simulink model "SimuLanzador"  (R2020b)
settings: Solver=VariableStepAuto  StartTime=0.0  StopTime=300  RelTol=1e-3
model workspace (MAT data in the model file):
  Ang0 = [0; 0; 0]
  VelAng0 = [0; 0; 0]
  altura = 3.5
  delta = 0.05
  mu = 0.01
  r = 2.25
  radio = 2.25
libraries: simulink_extras x5, sharedutil x5, sharedtransform x3, aerolibutil x2, aerolibbdyn x2, vrlib x1, simulink x1
settings Model: Creator=Sergio  LastModifiedBy=Sergio
settings SolverCC: ZeroCrossAlgorithm=Adaptive  AlgebraicLoopSolver=LineSearch

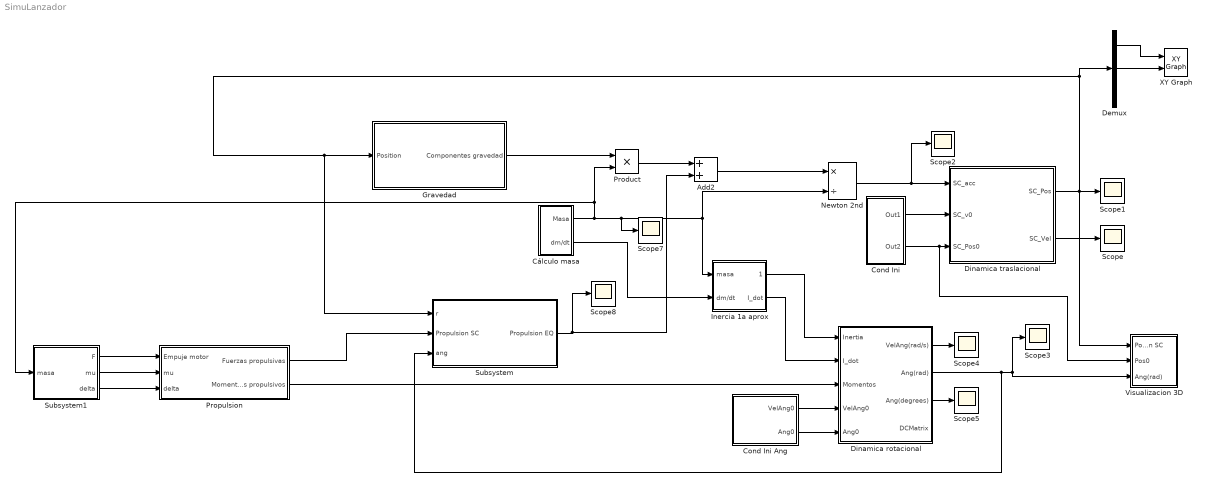
== system SimuLanzador ==
  Add2 : Sum
  Cond Ini : Subsystem  mask{v0=[0,0,0], Pos0=[1737100,0,0]}
  Cond Ini Ang : Subsystem  mask{VelAng0=[0,0,0], Ang0=[0,0,0]}
  Cálculo masa : Subsystem
  Demux : Demux  Outputs=3
  Dinamica rotacional : Subsystem
  Dinamica traslacional : Subsystem
  Gravedad : Subsystem
  Inercia 1a aprox : Subsystem
  Newton 2nd : Product  Inputs=*/
  Product : Product
  Propulsion : Subsystem
  Scope{,1..5,7..8} (8 alike) : Scope
  Subsystem : Subsystem
  Subsystem1 : Subsystem
  Visualizacion 3D : Subsystem
  XY Graph : simulink/Sinks/XY Graph  xmin=-2500000  xmax=2500000  ymin=-2500000  ymax=2500000  st=-1
  wires:
  Cond Ini/1(Out1) -> Dinamica traslacional/2(SC_v0)
  Cond Ini/2(Out2) -> Visualizacion 3D/2(Pos0), Dinamica traslacional/3(SC_Pos0)
  Newton 2nd/1 -> Scope2/1, Dinamica traslacional/1(SC_acc)
  Dinamica traslacional/2(SC_Vel) -> Scope/1
  Inercia 1a aprox/1(Inertia) -> Dinamica rotacional/1(Inertia)
  Dinamica rotacional/1(VelAng(rad/s)) -> Scope4/1
  Cond Ini Ang/1(VelAng0) -> Dinamica rotacional/4(VelAng0)
  Dinamica rotacional/3(Ang(degrees)) -> Scope5/1
  Product/1 -> Add2/1
  Gravedad/1(Componentes gravedad) -> Product/1
  Add2/1 -> Newton 2nd/1
  Subsystem/1(Propulsion EQ) -> Add2/2, Scope8/1
  Dinamica rotacional/2(Ang(rad)) -> Subsystem/3(ang), Scope3/1, Visualizacion 3D/3(Ang(rad))
  Inercia 1a aprox/2(I_dot) -> Dinamica rotacional/2(I_dot)
  Cálculo masa/2(dm/dt) -> Inercia 1a aprox/2(dm/dt)
  Cálculo masa/1(Masa) -> Scope7/1, Inercia 1a aprox/1(masa), Newton 2nd/2, Subsystem1/1(masa), Product/2
  Subsystem1/1(F) -> Propulsion/1(Empuje motor)
  Subsystem1/2(mu) -> Propulsion/2(mu)
  Subsystem1/3(delta) -> Propulsion/3(delta)
  Propulsion/1(Fuerzas propulsivas) -> Subsystem/2(Propulsion SC)
  Propulsion/2(Momentos propulsivos) -> Dinamica rotacional/3(Momentos)
  Dinamica traslacional/1(SC_Pos) -> Visualizacion 3D/1(Posicion SC), Demux/1, Subsystem/1(r), Gravedad/1(Position), Scope1/1
  Demux/1 -> XY Graph/1
  Cond Ini Ang/2(Ang0) -> Dinamica rotacional/5(Ang0)
  Demux/2 -> XY Graph/2

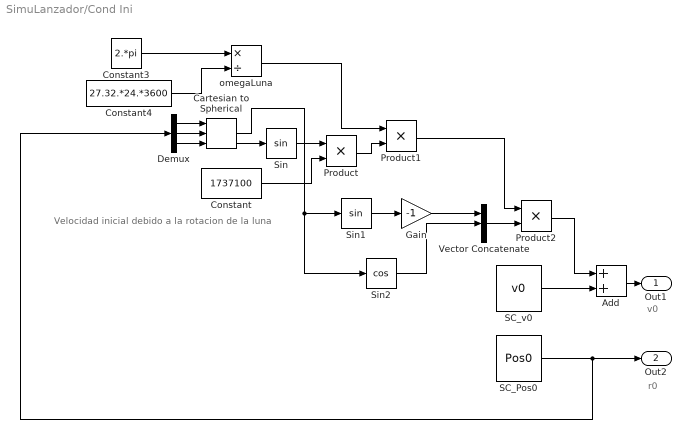
== system SimuLanzador/Cond Ini ==
  note: r0
  note: v0
  note: Velocidad inicial debido a la rotacion de la luna
  Add : Sum
  Cartesian to Spherical : simulink_extras/Transformations/Cartesian to Spherical
      settings: SourceProductBaseCode=SL
  Constant : Constant  Value=1737100
  Constant3 : Constant  Value=2.*pi
  Constant4 : Constant  Value=27.32.*24.*3600
  Demux : Demux  Outputs=3
  Gain : Gain  Gain=-1
  Product : Product
  Product1 : Product
  Product2 : Product
  SC_Pos0 : Constant  Value=Pos0  VectorParams1D=off
  SC_v0 : Constant  Value=v0  VectorParams1D=off
  Sin : Trigonometry
  Sin1 : Trigonometry
  Sin2 : Trigonometry  Operator=cos
  Vector Concatenate : Concatenate  NumInputs=3
  omegaLuna : Product  Inputs=*/
  Out1 : Outport
  Out2 : Outport  Port=2
  wires:
  Constant3/1 -> omegaLuna/1
  Product1/1 -> Product2/1
  Sin/1 -> Product/1
  Constant/1 -> Product/2
  Constant4/1 -> omegaLuna/2
  Product/1 -> Product1/2
  Sin1/1 -> Gain/1
  Product2/1 -> Add/1
  Cartesian to Spherical/2 -> Sin2/1, Sin1/1
  Vector Concatenate/1 -> Product2/2
  SC_Pos0/1 -> Out2/1, Demux/1
  Sin2/1 -> Vector Concatenate/2
  omegaLuna/1 -> Product1/1
  Demux/1 -> Cartesian to Spherical/1
  Demux/2 -> Cartesian to Spherical/2
  Gain/1 -> Vector Concatenate/1
  Demux/3 -> Cartesian to Spherical/3
  Cartesian to Spherical/3 -> Sin/1
  SC_v0/1 -> Add/2
  Add/1 -> Out1/1

== system SimuLanzador/Cond Ini Ang ==
  CIAng : Constant  Value=Ang0  VectorParams1D=off
  CIVelAng : Constant  Value=VelAng0  VectorParams1D=off
  VelAng0 : Outport
  Ang0 : Outport  Port=2
  wires:
  CIAng/1 -> Ang0/1
  CIVelAng/1 -> VelAng0/1

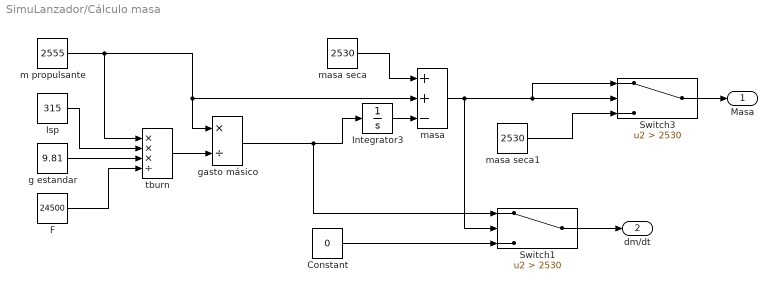
== system SimuLanzador/Cálculo masa ==
  Constant : Constant  Value=0
  F : Constant  Value=24500
  Integrator3 : Integrator
  Isp : Constant  Value=315
  Switch1 : Switch  Criteria=u2 > Threshold  Threshold=2530
  Switch3 : Switch  Criteria=u2 > Threshold  Threshold=2530
  g estandar : Constant  Value=9.81
  gasto másico : Product  Inputs=*/
  m propulsante : Constant  Value=2555
  masa : Sum  Inputs=++-
  masa seca : Constant  Value=2530
  masa seca1 : Constant  Value=2530
  tburn : Product  Inputs=***/
  Masa : Outport
  dm/dt : Outport  Port=2
  wires:
  masa seca1/1 -> Switch3/3
  g estandar/1 -> tburn/3
  gasto másico/1 -> Switch1/1, Integrator3/1
  m propulsante/1 -> tburn/1, masa/2, gasto másico/1
  tburn/1 -> gasto másico/2
  masa seca/1 -> masa/1
  masa/1 -> Switch1/2, Switch3/1, Switch3/2
  Isp/1 -> tburn/2
  Integrator3/1 -> masa/3
  Switch3/1 -> Masa/1
  Switch1/1 -> dm/dt/1
  F/1 -> tburn/4
  Constant/1 -> Switch1/3

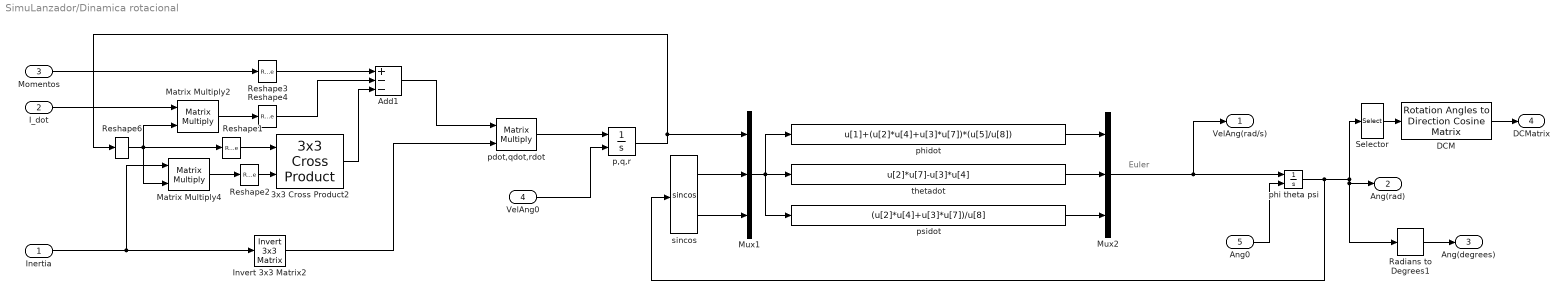
== system SimuLanzador/Dinamica rotacional ==
  note: Euler
  Inertia : Inport
  I_dot : Inport  Port=2
  Momentos : Inport  Port=3
  VelAng0 : Inport  Port=4
  Ang0 : Inport  Port=5
  3x3 Cross Product2 : sharedutil/3x3 Cross Product  aMode=aMode
      settings: SourceProductBaseCode=AE,PW,MT,UV,VE,VP
  Add1 : Sum  Inputs=+--
  DCM : sharedtransform/Rotation Angles to Direction Cosine Matrix  rotationOrder=ZYX  aMode=aMode
      settings: SourceProductBaseCode=AE,PW,MT,UV,VE,VP
  Invert 3x3 Matrix2 : aerolibutil/Invert  3x3 Matrix
  Matrix Multiply2 : Product  Multiplication=Matrix(*)
  Matrix Multiply4 : Product  Multiplication=Matrix(*)
  Mux1 : Mux  Inputs=[3 3 3]
  Mux2 : Mux  Inputs=3
  Radians to Degrees1 : simulink_extras/Transformations/Radians to Degrees
  Reshape{1..4} (4 alike) : Reshape  OutputDimensionality=Row vector (2-D)
  Reshape6 : Reshape  OutputDimensionality=Column vector (2-D)
  Selector : Selector  InputPortWidth=3  IndexOptions=Index vector (dialog)  Indices=[3 2 1]  OutputSizes=1
  p,q,r : Integrator  InitialConditionSource=external
  pdot,qdot,rdot : Product  Multiplication=Matrix(*)
  phi theta psi : Integrator  InitialConditionSource=external  WrapState=on
  phidot : Fcn  Expr=u[1]+(u[2]*u[4]+u[3]*u[7])*(u[5]/u[8])
  psidot : Fcn  Expr=(u[2]*u[4]+u[3]*u[7])/u[8]
  sincos : Trigonometry  Operator=sincos
  thetadot : Fcn  Expr=u[2]*u[7]-u[3]*u[4]
  VelAng(rad/s) : Outport
  Ang(rad) : Outport  Port=2
  Ang(degrees) : Outport  Port=3
  DCMatrix : Outport  Port=4
  wires:
  Invert 3x3 Matrix2/1 -> pdot,qdot,rdot/2
  Inertia/1 -> Matrix Multiply4/1, Invert 3x3 Matrix2/1
  Add1/1 -> pdot,qdot,rdot/1
  pdot,qdot,rdot/1 -> p,q,r/1
  I_dot/1 -> Matrix Multiply2/1
  3x3 Cross Product2/1 -> Add1/3
  Mux1/1 -> thetadot/1, phidot/1, psidot/1
  sincos/2 -> Mux1/3
  sincos/1 -> Mux1/2
  thetadot/1 -> Mux2/2
  phidot/1 -> Mux2/1
  psidot/1 -> Mux2/3
  Radians to Degrees1/1 -> Ang(degrees)/1
  Ang0/1 -> phi theta psi/2
  Mux2/1 -> phi theta psi/1, VelAng(rad/s)/1
  p,q,r/1 -> Reshape6/1, Mux1/1
  Reshape1/1 -> 3x3 Cross Product2/1
  Matrix Multiply4/1 -> Reshape2/1
  Reshape2/1 -> 3x3 Cross Product2/2
  Reshape3/1 -> Add1/1
  Momentos/1 -> Reshape3/1
  Matrix Multiply2/1 -> Reshape4/1
  Reshape4/1 -> Add1/2
  VelAng0/1 -> p,q,r/2
  Reshape6/1 -> Matrix Multiply2/2, Matrix Multiply4/2, Reshape1/1
  phi theta psi/1 -> Radians to Degrees1/1, Ang(rad)/1, Selector/1, sincos/1
  Selector/1 -> DCM/1
  DCM/1 -> DCMatrix/1

== system SimuLanzador/Dinamica traslacional ==
  SC_acc : Inport
  SC_v0 : Inport  Port=2
  SC_Pos0 : Inport  Port=3
  Add : Sum
  Add1 : Sum
  Integrator : Integrator
  Integrator1 : Integrator
  SC_Pos : Outport
  SC_Vel : Outport  Port=2
  wires:
  Add/1 -> SC_Vel/1, Integrator1/1
  Add1/1 -> SC_Pos/1
  SC_Pos0/1 -> Add1/2
  SC_acc/1 -> Integrator/1
  SC_v0/1 -> Add/2
  Integrator/1 -> Add/1
  Integrator1/1 -> Add1/1

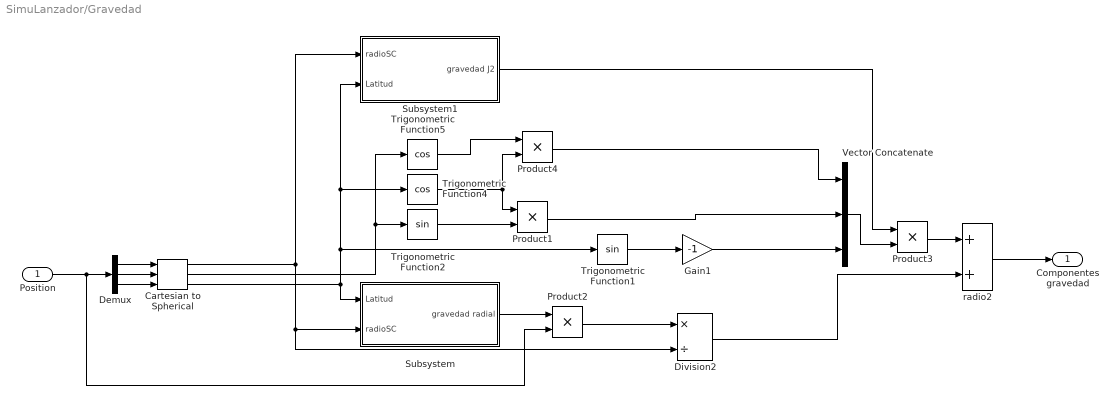
== system SimuLanzador/Gravedad ==
  Position : Inport
  Cartesian to Spherical : simulink_extras/Transformations/Cartesian to Spherical
      settings: SourceProductBaseCode=SL
  Demux : Demux  Outputs=3
  Division2 : Product  Inputs=*/
  Gain1 : Gain  Gain=-1
  Product{1..4} (4 alike) : Product
  Subsystem : Subsystem
  Subsystem1 : Subsystem
  Trigonometric Function1 : Trigonometry
  Trigonometric Function2 : Trigonometry
  Trigonometric Function4 : Trigonometry  Operator=cos
  Trigonometric Function5 : Trigonometry  Operator=cos
  Vector Concatenate : Concatenate  NumInputs=3
  radio2 : Sum
  Componentes gravedad : Outport
  wires:
  Position/1 -> Product2/2, Demux/1
  Cartesian to Spherical/1 -> Subsystem/2(radioSC), Division2/2, Subsystem1/1(radioSC)
  Product2/1 -> Division2/1
  Demux/2 -> Cartesian to Spherical/2
  Demux/1 -> Cartesian to Spherical/1
  Demux/3 -> Cartesian to Spherical/3
  Subsystem/1(gravedad radial) -> Product2/1
  Division2/1 -> radio2/2
  radio2/1 -> Componentes gravedad/1
  Product3/1 -> radio2/1
  Vector Concatenate/1 -> Product3/2
  Subsystem1/1(gravedad J2) -> Product3/1
  Cartesian to Spherical/3 -> Subsystem/1(Latitud), Trigonometric Function1/1, Trigonometric Function4/1, Subsystem1/2(Latitud)
  Trigonometric Function5/1 -> Product4/1
  Trigonometric Function2/1 -> Product1/2
  Product1/1 -> Vector Concatenate/2
  Trigonometric Function4/1 -> Product4/2, Product1/1
  Cartesian to Spherical/2 -> Trigonometric Function5/1, Trigonometric Function2/1
  Product4/1 -> Vector Concatenate/1
  Gain1/1 -> Vector Concatenate/3
  Trigonometric Function1/1 -> Gain1/1

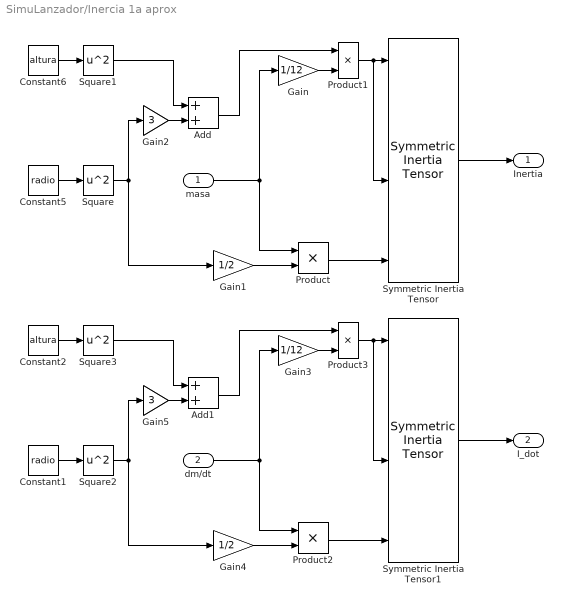
== system SimuLanzador/Inercia 1a aprox ==
  masa : Inport
  dm/dt : Inport  Port=2
  Add : Sum
  Add1 : Sum
  Constant1 : Constant  Value=radio
  Constant2 : Constant  Value=altura
  Constant5 : Constant  Value=radio
  Constant6 : Constant  Value=altura
  Gain : Gain  Gain=1/12
  Gain1 : Gain  Gain=1/2
  Gain2 : Gain  Gain=3
  Gain3 : Gain  Gain=1/12
  Gain4 : Gain  Gain=1/2
  Gain5 : Gain  Gain=3
  Product{,1..3} (4 alike) : Product
  Square{,1..3} (4 alike) : Math  Operator=square  SaturateOnIntegerOverflow=on
  Symmetric Inertia Tensor : aerolibbdyn/Symmetric Inertia Tensor
      settings: SourceProductBaseCode=AE
  Symmetric Inertia Tensor1 : aerolibbdyn/Symmetric Inertia Tensor
      settings: SourceProductBaseCode=AE
  Inertia : Outport
  I_dot : Outport  Port=2
  wires:
  Gain2/1 -> Add/2
  Square1/1 -> Add/1
  Product/1 -> Symmetric Inertia Tensor/6
  masa/1 -> Gain/1, Product/1
  Gain/1 -> Product1/2
  Symmetric Inertia Tensor/1 -> Inertia/1
  Square/1 -> Gain2/1, Gain1/1
  Add/1 -> Product1/1
  Product1/1 -> Symmetric Inertia Tensor/4, Symmetric Inertia Tensor/1
  Gain1/1 -> Product/2
  Constant5/1 -> Square/1
  Constant6/1 -> Square1/1
  Constant1/1 -> Square2/1
  Square2/1 -> Gain5/1, Gain4/1
  Constant2/1 -> Square3/1
  Square3/1 -> Add1/1
  Product3/1 -> Symmetric Inertia Tensor1/4, Symmetric Inertia Tensor1/1
  Gain5/1 -> Add1/2
  Gain3/1 -> Product3/2
  Gain4/1 -> Product2/2
  Product2/1 -> Symmetric Inertia Tensor1/6
  Add1/1 -> Product3/1
  dm/dt/1 -> Gain3/1, Product2/1
  Symmetric Inertia Tensor1/1 -> I_dot/1

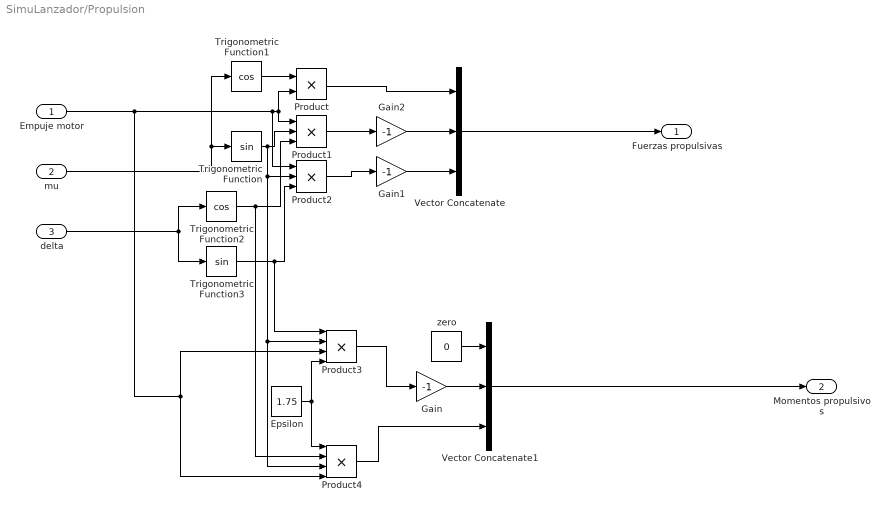
== system SimuLanzador/Propulsion ==
  Empuje motor : Inport
  mu : Inport  Port=2
  delta : Inport  Port=3
  Epsilon : Constant  Value=1.75
  Gain : Gain  Gain=-1
  Gain1 : Gain  Gain=-1
  Gain2 : Gain  Gain=-1
  Product : Product
  Product1 : Product  Inputs=3
  Product2 : Product  Inputs=3
  Product3 : Product  Inputs=4
  Product4 : Product  Inputs=4
  Trigonometric Function : Trigonometry
  Trigonometric Function1 : Trigonometry  Operator=cos
  Trigonometric Function2 : Trigonometry  Operator=cos
  Trigonometric Function3 : Trigonometry
  Vector Concatenate : Concatenate  NumInputs=3
  Vector Concatenate1 : Concatenate  NumInputs=3
  zero : Constant  Value=0
  Fuerzas propulsivas : Outport
  Momentos propulsivos : Outport  Port=2
  wires:
  Product4/1 -> Vector Concatenate1/3
  zero/1 -> Vector Concatenate1/1
  Trigonometric Function1/1 -> Product/1
  delta/1 -> Trigonometric Function2/1, Trigonometric Function3/1
  Trigonometric Function/1 -> Product4/3, Product3/2, Product2/2, Product1/2
  Empuje motor/1 -> Product4/4, Product3/3, Product2/1, Product/2, Product1/1
  Trigonometric Function3/1 -> Product3/1, Product2/3
  mu/1 -> Trigonometric Function/1, Trigonometric Function1/1
  Trigonometric Function2/1 -> Product4/2, Product1/3
  Epsilon/1 -> Product3/4, Product4/1
  Product/1 -> Vector Concatenate/1
  Vector Concatenate/1 -> Fuerzas propulsivas/1
  Vector Concatenate1/1 -> Momentos propulsivos/1
  Product2/1 -> Gain1/1
  Product1/1 -> Gain2/1
  Gain2/1 -> Vector Concatenate/2
  Gain1/1 -> Vector Concatenate/3
  Gain/1 -> Vector Concatenate1/2
  Product3/1 -> Gain/1

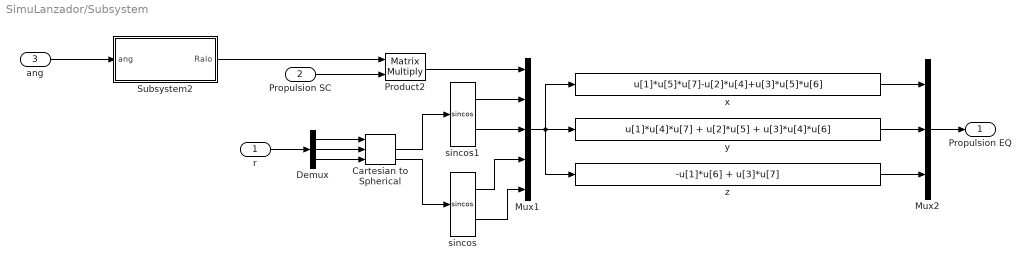
== system SimuLanzador/Subsystem ==
  r : Inport
  Propulsion SC : Inport  Port=2
  ang : Inport  Port=3
  Cartesian to Spherical : simulink_extras/Transformations/Cartesian to Spherical
      settings: SourceProductBaseCode=SL
  Demux : Demux  Outputs=3
  Mux1 : Mux  Inputs=[3 1 1 1 1]
  Mux2 : Mux  Inputs=3
  Product2 : Product  Multiplication=Matrix(*)
  Subsystem2 : Subsystem
  sincos : Trigonometry  Operator=sincos
  sincos1 : Trigonometry  Operator=sincos
  x : Fcn  Expr=u[1]*u[5]*u[7]-u[2]*u[4]+u[3]*u[5]*u[6]
  y : Fcn  Expr=u[1]*u[4]*u[7] + u[2]*u[5] + u[3]*u[4]*u[6]
  z : Fcn  Expr=-u[1]*u[6] + u[3]*u[7]
  Propulsion EQ : Outport
  wires:
  Propulsion SC/1 -> Product2/2
  Demux/3 -> Cartesian to Spherical/3
  r/1 -> Demux/1
  Demux/2 -> Cartesian to Spherical/2
  Demux/1 -> Cartesian to Spherical/1
  sincos/2 -> Mux1/5
  z/1 -> Mux2/3
  x/1 -> Mux2/1
  y/1 -> Mux2/2
  Product2/1 -> Mux1/1
  Mux1/1 -> y/1, x/1, z/1
  sincos/1 -> Mux1/4
  sincos1/2 -> Mux1/3
  sincos1/1 -> Mux1/2
  Cartesian to Spherical/2 -> sincos1/1
  Cartesian to Spherical/3 -> sincos/1
  Mux2/1 -> Propulsion EQ/1
  Subsystem2/1(Ralo) -> Product2/1
  ang/1 -> Subsystem2/1(ang)

== system SimuLanzador/Subsystem1 ==
  masa : Inport
  Constant : Constant  Value=0
  Constant2 : Constant  Value=0.00001
  Empuje : Constant  Value=24500
  Switch : Switch  Criteria=u2 > Threshold  Threshold=2530
  delta(rad) : Sin  Amplitude=0.01  Frequency=0.001  SampleTime=0
  mu(rad) : Sin  Amplitude=0.05  Frequency=0.001  SampleTime=0
  F : Outport
  mu : Outport  Port=2
  delta : Outport  Port=3
  wires:
  masa/1 -> Switch/2
  Empuje/1 -> Switch/1
  Constant/1 -> delta/1, Switch/3
  Switch/1 -> F/1
  Constant2/1 -> mu/1

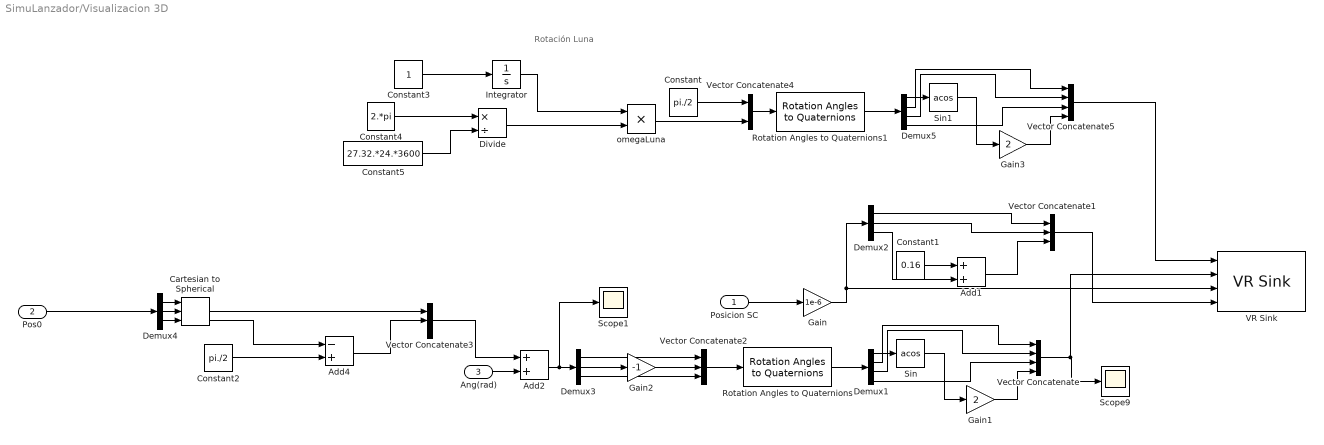
== system SimuLanzador/Visualizacion 3D ==
  note: Rotación Luna
  Posicion SC : Inport
  Pos0 : Inport  Port=2
  Ang(rad) : Inport  Port=3
  Add1 : Sum
  Add2 : Sum
  Add4 : Sum  Inputs=-+
  Cartesian to Spherical : simulink_extras/Transformations/Cartesian to Spherical
      settings: SourceProductBaseCode=SL
  Constant : Constant  Value=pi./2
  Constant1 : Constant  Value=0.16
  Constant2 : Constant  Value=pi./2
  Constant3 : Constant
  Constant4 : Constant  Value=2.*pi
  Constant5 : Constant  Value=27.32.*24.*3600
  Demux1 : Demux
  Demux2 : Demux  Outputs=3
  Demux3 : Demux  Outputs=3
  Demux4 : Demux  Outputs=3
  Demux5 : Demux
  Divide : Product  Inputs=*/
  Gain : Gain  Gain=1e-6
  Gain1 : Gain  Gain=2
  Gain2 : Gain  Gain=-1
  Gain3 : Gain  Gain=2
  Integrator : Integrator
  Rotation Angles to Quaternions : sharedtransform/Rotation Angles to Quaternions  rotationOrder=ZYZ  aMode=aMode
      settings: SourceProductBaseCode=AE,PW,MT,UV,VE,VP
  Rotation Angles to Quaternions1 : sharedtransform/Rotation Angles to Quaternions  rotationOrder=XYZ  aMode=aMode
      settings: SourceProductBaseCode=AE,PW,MT,UV,VE,VP
  Scope1 : Scope
  Scope9 : Scope
  Sin : Trigonometry  Operator=acos
  Sin1 : Trigonometry  Operator=acos
  VR Sink : vrlib/VR Sink  InstantiateOnLoad=on  SampleTime=0.1  ViewEnable=on  RemoteChange=off  RemoteView=off  FieldsWritten=MOON.rotation.4.1.1.double#SC.rotation.4.1.1.double#SC.translation.3.1.1.double#Lanzamiento.position.3.1.1.double  WorldFileName=3dprueba3.x3d  AutoView=off  VideoDimensions=[]  AllowVariableSize=off
  Vector Concatenate : Concatenate  NumInputs=4
  Vector Concatenate{1..4} (4 alike) : Concatenate  NumInputs=3
  Vector Concatenate5 : Concatenate  NumInputs=4
  omegaLuna : Product
  wires:
  Constant1/1 -> Add1/1
  Demux2/2 -> Vector Concatenate1/2
  Demux1/3 -> Vector Concatenate/2
  Vector Concatenate1/1 -> VR Sink/4
  Demux1/1 -> Sin/1
  Demux2/3 -> Add1/2
  Add1/1 -> Vector Concatenate1/3
  Gain/1 -> VR Sink/3, Demux2/1
  Gain1/1 -> Vector Concatenate/4
  Demux1/4 -> Vector Concatenate/3
  Sin/1 -> Gain1/1
  Demux2/1 -> Vector Concatenate1/1
  Rotation Angles to Quaternions/1 -> Demux1/1
  Demux1/2 -> Vector Concatenate/1
  Posicion SC/1 -> Gain/1
  Vector Concatenate2/1 -> Rotation Angles to Quaternions/1
  Demux3/1 -> Vector Concatenate2/1
  Demux3/3 -> Vector Concatenate2/3
  Vector Concatenate/1 -> VR Sink/2, Scope9/1
  Demux4/2 -> Cartesian to Spherical/2
  Demux4/3 -> Cartesian to Spherical/3
  Demux4/1 -> Cartesian to Spherical/1
  Vector Concatenate3/1 -> Add2/1
  Cartesian to Spherical/3 -> Add4/1
  Pos0/1 -> Demux4/1
  Add4/1 -> Vector Concatenate3/2
  Add2/1 -> Scope1/1, Demux3/1
  Ang(rad)/1 -> Add2/2
  Vector Concatenate5/1 -> VR Sink/1
  Integrator/1 -> omegaLuna/1
  Constant/1 -> Vector Concatenate4/1
  Rotation Angles to Quaternions1/1 -> Demux5/1
  omegaLuna/1 -> Vector Concatenate4/3
  Gain3/1 -> Vector Concatenate5/4
  Demux5/3 -> Vector Concatenate5/2
  Demux5/4 -> Vector Concatenate5/3
  Constant3/1 -> Integrator/1
  Demux5/2 -> Vector Concatenate5/1
  Vector Concatenate4/1 -> Rotation Angles to Quaternions1/1
  Divide/1 -> omegaLuna/2
  Demux5/1 -> Sin1/1
  Sin1/1 -> Gain3/1
  Constant4/1 -> Divide/1
  Constant5/1 -> Divide/2
  Constant2/1 -> Add4/2
  Gain2/1 -> Vector Concatenate2/2
  Demux3/2 -> Gain2/1
  Cartesian to Spherical/2 -> Vector Concatenate3/1

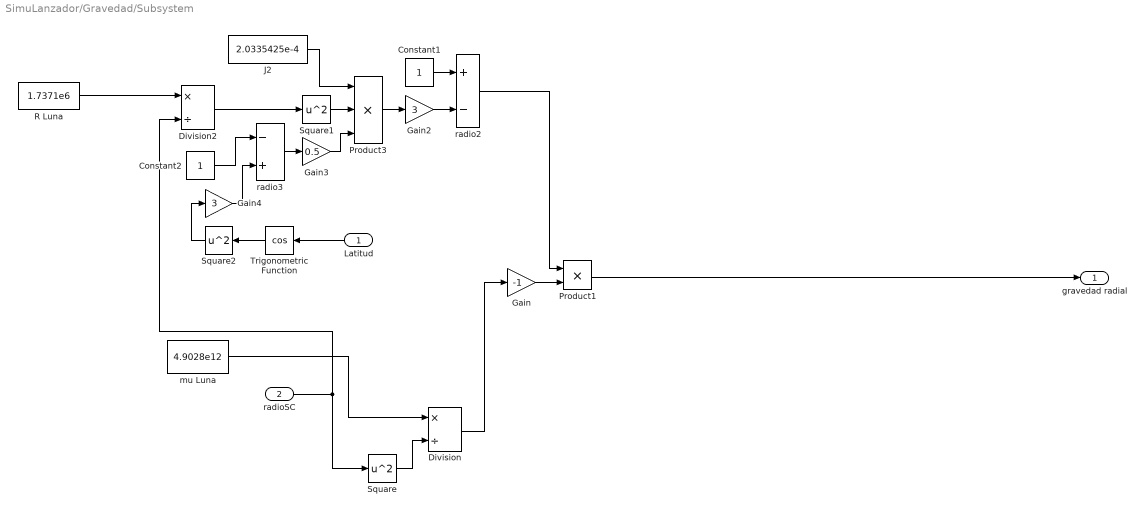
== system SimuLanzador/Gravedad/Subsystem ==
  Latitud : Inport
  radioSC : Inport  Port=2
  Constant1 : Constant
  Constant2 : Constant
  Division : Product  Inputs=*/
  Division2 : Product  Inputs=*/
  Gain : Gain  Gain=-1
  Gain2 : Gain  Gain=3
  Gain3 : Gain  Gain=0.5
  Gain4 : Gain  Gain=3
  J2 : Constant  Value=2.0335425e-4
  Product1 : Product
  Product3 : Product  Inputs=3
  R Luna : Constant  Value=1.7371e6
  Square : Math  Operator=square  SaturateOnIntegerOverflow=on
  Square1 : Math  Operator=square  SaturateOnIntegerOverflow=on
  Square2 : Math  Operator=square  SaturateOnIntegerOverflow=on
  Trigonometric Function : Trigonometry  Operator=cos
  mu Luna : Constant  Value=4.9028e12
  radio2 : Sum  Inputs=+-
  radio3 : Sum  Inputs=-+
  gravedad radial : Outport
  wires:
  radio2/1 -> Product1/1
  R Luna/1 -> Division2/1
  mu Luna/1 -> Division/1
  Gain3/1 -> Product3/3
  radioSC/1 -> Square/1, Division2/2
  J2/1 -> Product3/1
  Division2/1 -> Square1/1
  Square1/1 -> Product3/2
  Division/1 -> Gain/1
  Constant1/1 -> radio2/1
  Latitud/1 -> Trigonometric Function/1
  Product3/1 -> Gain2/1
  Gain2/1 -> radio2/2
  Trigonometric Function/1 -> Square2/1
  Gain/1 -> Product1/2
  radio3/1 -> Gain3/1
  Square/1 -> Division/2
  Constant2/1 -> radio3/1
  Square2/1 -> Gain4/1
  Gain4/1 -> radio3/2
  Product1/1 -> gravedad radial/1

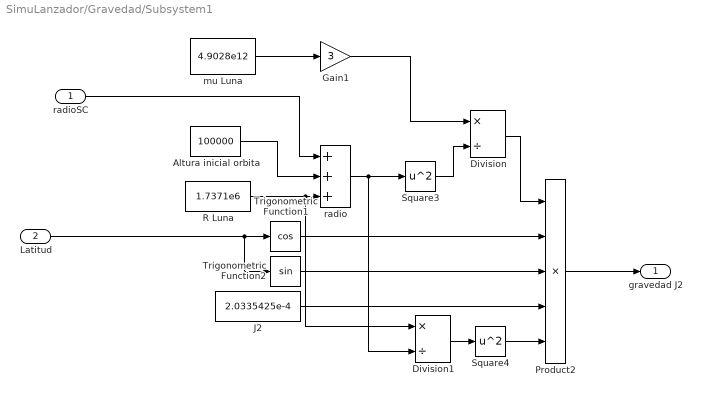
== system SimuLanzador/Gravedad/Subsystem1 ==
  radioSC : Inport
  Latitud : Inport  Port=2
  Altura inicial orbita : Constant  Value=100000
  Division : Product  Inputs=*/
  Division1 : Product  Inputs=*/
  Gain1 : Gain  Gain=3
  J2 : Constant  Value=2.0335425e-4
  Product2 : Product  Inputs=5
  R Luna : Constant  Value=1.7371e6
  Square3 : Math  Operator=square  SaturateOnIntegerOverflow=on
  Square4 : Math  Operator=square  SaturateOnIntegerOverflow=on
  Trigonometric Function1 : Trigonometry  Operator=cos
  Trigonometric Function2 : Trigonometry
  mu Luna : Constant  Value=4.9028e12
  radio : Sum  Inputs=+++
  gravedad J2 : Outport
  wires:
  mu Luna/1 -> Gain1/1
  radioSC/1 -> radio/1
  R Luna/1 -> Division1/1, radio/3
  radio/1 -> Division1/2, Square3/1
  Division/1 -> Product2/1
  Square3/1 -> Division/2
  Altura inicial orbita/1 -> radio/2
  Gain1/1 -> Division/1
  Latitud/1 -> Trigonometric Function2/1, Trigonometric Function1/1
  Trigonometric Function1/1 -> Product2/2
  Trigonometric Function2/1 -> Product2/3
  J2/1 -> Product2/4
  Square4/1 -> Product2/5
  Division1/1 -> Square4/1
  Product2/1 -> gravedad J2/1

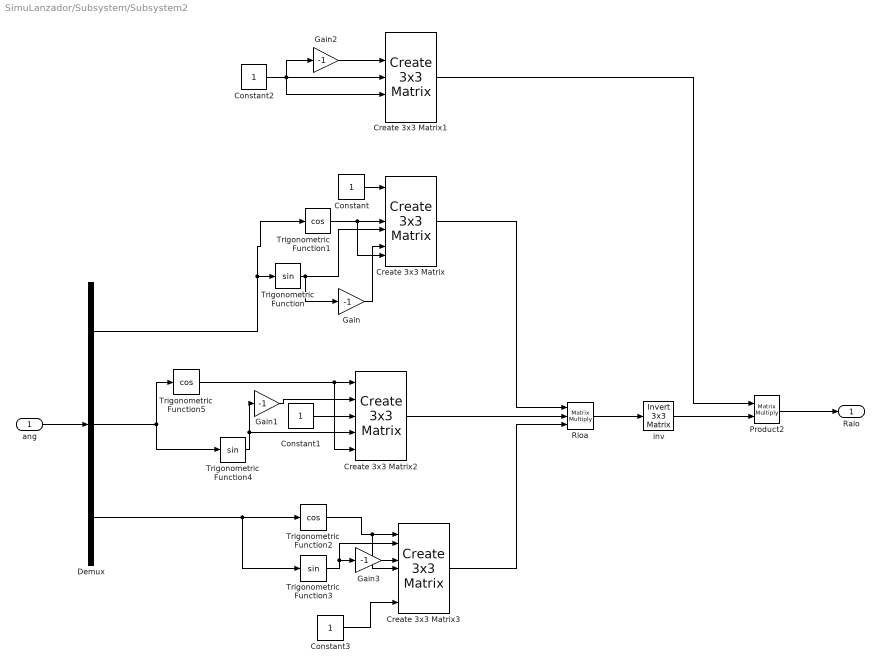
== system SimuLanzador/Subsystem/Subsystem2 ==
  ang : Inport
  Constant{,1..3} (4 alike) : Constant
  Create 3x3 Matrix{,1..3} (4 alike) : sharedutil/Create 3x3 Matrix  aMode=aMode
      settings: SourceProductBaseCode=AE,PW,MT,UV,VE,VP
  Demux : Demux  Outputs=3
  Gain{,1..3} (4 alike) : Gain  Gain=-1
  Product2 : Product  Multiplication=Matrix(*)
  Rloa : Product  Inputs=3  Multiplication=Matrix(*)
  Trigonometric Function : Trigonometry
  Trigonometric Function1 : Trigonometry  Operator=cos
  Trigonometric Function2 : Trigonometry  Operator=cos
  Trigonometric Function3 : Trigonometry
  Trigonometric Function4 : Trigonometry
  Trigonometric Function5 : Trigonometry  Operator=cos
  inv : aerolibutil/Invert  3x3 Matrix
  Ralo : Outport
  wires:
  Create 3x3 Matrix2/1 -> Rloa/2
  Constant3/1 -> Create 3x3 Matrix3/9
  Gain3/1 -> Create 3x3 Matrix3/4
  Trigonometric Function3/1 -> Gain3/1, Create 3x3 Matrix3/2
  Create 3x3 Matrix3/1 -> Rloa/3
  Trigonometric Function2/1 -> Create 3x3 Matrix3/5, Create 3x3 Matrix3/1
  ang/1 -> Demux/1
  Trigonometric Function/1 -> Create 3x3 Matrix/6, Gain/1
  Constant/1 -> Create 3x3 Matrix/1
  Trigonometric Function1/1 -> Create 3x3 Matrix/9, Create 3x3 Matrix/5
  Demux/1 -> Trigonometric Function1/1, Trigonometric Function/1
  Create 3x3 Matrix/1 -> Rloa/1
  Demux/3 -> Trigonometric Function3/1, Trigonometric Function2/1
  Constant1/1 -> Create 3x3 Matrix2/5
  Demux/2 -> Trigonometric Function4/1, Trigonometric Function5/1
  Trigonometric Function4/1 -> Create 3x3 Matrix2/7, Gain1/1
  Gain1/1 -> Create 3x3 Matrix2/3
  Trigonometric Function5/1 -> Create 3x3 Matrix2/9, Create 3x3 Matrix2/1
  Gain/1 -> Create 3x3 Matrix/8
  Constant2/1 -> Create 3x3 Matrix1/7, Create 3x3 Matrix1/5, Gain2/1
  Create 3x3 Matrix1/1 -> Product2/1
  Product2/1 -> Ralo/1
  inv/1 -> Product2/2
  Rloa/1 -> inv/1
  Gain2/1 -> Create 3x3 Matrix1/3
